simulink model "solar"  (Simulink 7.5)
settings: Solver=ode23t  StartTime=0.0  StopTime=50  RelTol=1e-3
libraries: nesl_utility x3, fl_lib x2, elec_lib x2
settings Model: Creator=nrqm  LastModifiedBy=nrqm

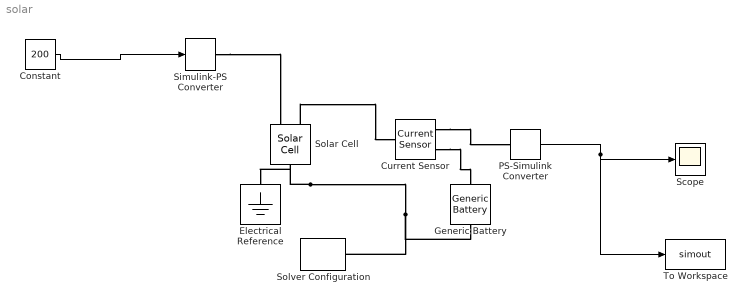
== system solar ==
  Constant : Constant  Value=200  OutDataType=fixdt(1, 16)  OutScaling=2^0
  Current Sensor : fl_lib/Electrical/Electrical Sensors/Current Sensor  DialogController=NetworkEngine.DynNeDlgSource  SystemSampleTime=-1  i1_Log=off  v1_Log=off  LocalVarNames=|i1|v1  LocalVarDescs=|i1|v1  LocalVarLogging=[0 0]
  Electrical Reference : fl_lib/Electrical/Electrical Elements/Electrical Reference  DialogController=NetworkEngine.DynNeDlgSource  SystemSampleTime=-1  i_Log=off  LocalVarNames=|i  LocalVarDescs=|i  LocalVarLogging=0
  Generic Battery : elec_lib/Sources/Generic Battery  DialogController=NetworkEngine.DynNeDlgSource  SystemSampleTime=-1  Vnom=3 V  R1=2 Ohm  prm_AH=2  AH=4 hr*A  AH0=1 hr*A  V1=1.8 V  AH1=0.2 hr*A  prm_R2=1  R2=2e+3 Ohm  LocalVarLogging=[]
  PS-Simulink Converter : nesl_utility/PS-Simulink Converter  DialogController=NetworkEngine.DynNeUtilDlgSource  SystemSampleTime=-1  PhysicalDomain=network_engine_domain  LeftPortType=input  RightPortType=output  SubClassName=ps_output  Unit=1  AffineConversion=off
  Scope : Scope
  Simulink-PS Converter : nesl_utility/Simulink-PS Converter  DialogController=NetworkEngine.DynNeUtilDlgSource  SystemSampleTime=-1  PhysicalDomain=network_engine_domain  LeftPortType=input  RightPortType=output  SubClassName=ps_input  Unit=1  AffineConversion=off  InputFilterTimeConstant=.001  UdotUserProvided=0
  Solar Cell : elec_lib/Sources/Solar Cell  DialogController=NetworkEngine.DynNeDlgSource  SystemSampleTime=-1  prm=1  Isc=3.8 A  Voc=21.1 V  Is=1.296e-15 A  Is2=0 A  Iph=7.34 A  Ir0=1000 W/m^2  ec=1.5  N2=2  Rs=0 Ohm  Rp=Inf Ohm  TIPH1=0 1/K  EG=1.11 eV  TXIS1=3  TXIS2=3  TRS1=0  TRP1=0  TFIXED=303 K  Tmeas=303 K  LocalVarLogging=[]
  Solver Configuration : nesl_utility/Solver Configuration  DialogController=NetworkEngine.DynNeUtilDlgSource  SystemSampleTime=-1  PhysicalDomain=network_engine_domain  LeftPortType=input  RightPortType=generic  SubClassName=solver  Accelerate=off  Profile=off  ResidualTolerance=1e-9  MaxNonlinIter=3  MaxModeIter=2  DoFixedCost=off  UseLocalSampling=off  DoDC=off  LinearAlgebra=Sparse  LocalSolverSampleTime=.001  LocalSolverChoice=NE_BACKWARD_EULER_ADVANCER  UseLocalSolver=off
  To Workspace : ToWorkspace  VariableName=simout  SampleTime=-1  SaveFormat=Structure
  wires:
  PS-Simulink Converter/1 -> Scope/1, To Workspace/1
  Constant/1 -> Simulink-PS Converter/1
  connections:
  Current Sensor/RConn1 -- PS-Simulink Converter/LConn1
  Simulink-PS Converter/RConn1 -- Solar Cell/LConn1
  Solar Cell/RConn1 -- Electrical Reference/LConn1 -- Solver Configuration/RConn1 -- Generic Battery/RConn1
  Solar Cell/LConn2 -- Current Sensor/LConn1
  Current Sensor/RConn2 -- Generic Battery/LConn1
